simulink model "CartPoleSwingUp_Sim"  (R2019a)
settings: Solver=ode3  StartTime=0.0  StopTime=6  FixedStep=tstep  RelTol=1e-3
InitFcn:
  | initSim;
StopFcn:
  | plotSimSolution;
undefined symbols (not defined in the file or in its folder): m, par, problem, tstep
settings Model: Creator=yn15  LastModifiedBy=Yuanb
settings DataIOCC: ReturnWorkspaceOutputs=off
settings OptimizationCC: LifeSpan=inf
settings DebuggingCC: SFUnexpectedBacktrackingDiag=warning  SFNoUnconditionalDefaultTransitionDiag=warning  SFExecutionAtInitializationDiag=none  ArithmeticOperatorsInVariantConditions=warning
settings SFSimCC: SimUseLocalCustomCode=off
settings RTWCC: RTWUseLocalCustomCode=off
settings CodeAppCC: StateflowObjectComments=on
settings GRTTargetCC: TargetLangStandard=C89/C90 (ANSI)
settings ConfigComp: CovMetricSettings=dw  CovHtmlReporting=on  CovSaveCumulativeToWorkspaceVar=on  CovSaveSingleToWorkspaceVar=on  CovExternalEMLEnable=off

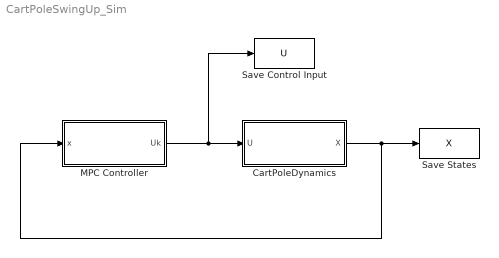
== system CartPoleSwingUp_Sim ==
  CartPoleDynamics : Subsystem
  "MPC Controller " : Subsystem
  Save Control Input : ToWorkspace  VariableName=U  SampleTime=-1
      settings: Save2DSignal=2-D array (concatenate along first dimension)
  Save States : ToWorkspace  VariableName=X  SampleTime=-1
  wires:
  "MPC Controller "/1(Uk) -> CartPoleDynamics/1(U), Save Control Input/1
  CartPoleDynamics/1(X) -> "MPC Controller "/1(x), Save States/1

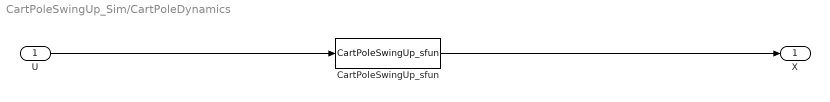
== system CartPoleSwingUp_Sim/CartPoleDynamics ==
  U : Inport
  CartPoleSwingUp_sfun : S-Function  FunctionName=CartPoleSwingUp_sfun  Parameters=par;problem.states.x0  SFunctionDeploymentMode=off  EnableBusSupport=off
  X : Outport
  wires:
  CartPoleSwingUp_sfun/1 -> X/1
  U/1 -> CartPoleSwingUp_sfun/1

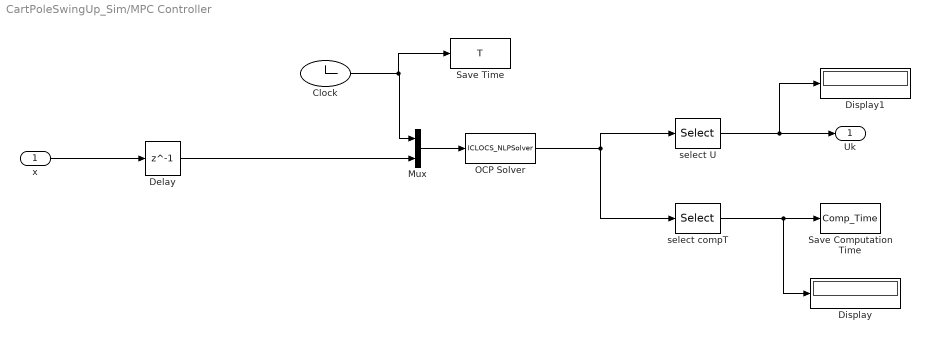
== system CartPoleSwingUp_Sim/MPC Controller  ==
  x : Inport
  Clock : Clock
  Delay : Delay  DelayLength=1  InitialCondition=[problem.states.x0]
  Display : Display
  Display1 : Display
  Mux : Mux  Inputs=2
  OCP Solver : MATLABFcn  MATLABFcn=ICLOCS_NLPSolver  OutputDimensions=m+2
  "Save Computation Time " : ToWorkspace  VariableName=Comp_Time  SampleTime=tstep
      settings: Save2DSignal=2-D array (concatenate along first dimension)
  Save Time : ToWorkspace  VariableName=T  SampleTime=-1
      settings: Save2DSignal=2-D array (concatenate along first dimension)
  select U : Selector  IndexOptions=Index vector (dialog)  Indices=3:m+2  OutputSizes=1
  select compT : Selector  IndexOptions=Index vector (dialog)  Indices=2  OutputSizes=1
  Uk : Outport
  wires:
  select U/1 -> Display1/1, Uk/1
  x/1 -> Delay/1
  OCP Solver/1 -> select compT/1, select U/1
  Clock/1 -> Save Time/1, Mux/1
  Mux/1 -> OCP Solver/1
  Delay/1 -> Mux/2
  select compT/1 -> Display/1, "Save Computation Time "/1
